simulink model "bus_roadtest_v3"  (R2018a)
settings: Solver=ode3  StartTime=0.0  StopTime=inf  FixedStep=0.01  RelTol=1e-3  EnableMultiTasking=on
PostLoadFcn:
  | , if any(exist('dsrtsu_mdlpostloadfcn', 'file') == [2, 3, 6]), try dsrtsu_mdlpostloadfcn('Execute', bdroot); catch fprintf('Error in PostLoadFcn (dsrtsu_mdlpostloadfcn) for model "%s":\n %s\n', bdroot, lasterr); end, end,
InitFcn:
  | bus_roadtest_v3_initial
values from neighbouring files (symbols this model uses):
  ay_max = 2    [Ini.m]
  delta_t = 0.01    [Ini.m]
  end_left_pass = 1    [Ini.m]
  end_right_pass = 0    [Ini.m]
  finish_node_id = length(Map_data(:,1))    [Ini.m]
  forward_length = 15    [Ini.m]
  gamma = sqrt(N_xaug+lambda)    [bus_roadtest_v3_initial.m]
  k_safe = 1    [Ini.m]
  nodes = nodes(1:index_node,:)    [Ini.m]
  rmin = 10    [Ini.m]
  segments = zeros(length(xy_ends_Pos(:,1)),3)    [Ini.m]
  start_node_id = 1    [Ini.m]
  Ts = 0.01    [bus_roadtest_v3_initial.m]
  Veh_CG = [0.5, 0.2]    [Ini.m]
  Veh_size = [1.99986,6.09558]    [Ini.m]
  vmax = 6    [Ini.m]
  weight = [weight_0,weight_0_cov,weight_i]    [bus_roadtest_v3_initial.m]
undefined symbols (not defined in the file or in its folder): Brake_table, DiscIntNeverNeededParam, Map_data, R, REF_GPS_RFS, Steer_gain_table, T
libraries: rtican x71, simulink x26, rti1401lib_adc_type4 x8, rti1401lib_dio_type4 x1
(part 18 of 18)

== matlab function bus_roadtest_v3/Target_planner/EndPointDecision1 ==
  data: x input; y input; End_x output; Path_x_0 input size=length(nodes(:,1)); Path_y_0 input size=length(nodes(:,1)); forward_length input; End_y output; path_length output
function [End_x,End_y,path_length] = EndPointDecision(x,y,Path_x_0,Path_y_0,forward_length)

% x = Vehicle_state(1,1); %vehicle global coordinate
% y = Vehicle_state(2,1);

Path_x = Path_x_0;
Path_y = Path_y_0;

%% Target plan
Path_RES_0 = zeros(20000,2);
Path_RES_0_1 = zeros(20000,2);
Res = 0.1;
count = 0;
count_1 = 0;
break_count = 0;
target_k = floor(forward_length/Res);

%找出切成10公分之投影點
Length_1 = ((Path_x(2)-Path_x(1))^2+(Path_y(2)-Path_y(1))^2)^0.5;
ang_1 = atan2(Path_y(2)-Path_y(1),Path_x(2)-Path_x(1));
if Length_1 > Res
    for j = 1:round(Length_1/Res)
        Path_RES_0_1(j,1) = Path_x(1) + (j-1)*Res*cos(ang_1);
        Path_RES_0_1(j,2) = Path_y(1) + (j-1)*Res*sin(ang_1);
        count_1 = j;
    end
else
    Path_RES_0_1(1,1) = Path_x(1);
    Path_RES_0_1(1,2) = Path_y(1);
    count_1 = 1;
end
Path_RES_1 = Path_RES_0_1((1:count_1),:);
ob_distance = (x-Path_RES_1(:,1)).^2 + (y - Path_RES_1(:,2)).^2;
[none,v_i] = min(ob_distance);
x_ob = Path_RES_1(v_i,1);
y_ob = Path_RES_1(v_i,2);
o_i = count_1-v_i;

if numel(Path_x(:,1))-2 >=1
    for i = 1:numel(Path_x(:,1))-2
        k = i+1;
        if break_count == 0
            Length = ((Path_x(k+1)-Path_x(k))^2+(Path_y(k+1)-Path_y(k))^2)^0.5;
            ang = atan2(Path_y(k+1)-Path_y(k),Path_x(k+1)-Path_x(k));
            if Length >= Res
                index_j = round(Length/Res);
                for j = 1:index_j
                    Path_RES_0(j+count,1) = Path_x(k) + (j-1)*Res*cos(ang);
                    Path_RES_0(j+count,2) = Path_y(k) + (j-1)*Res*sin(ang);
                end
                count = count + index_j;
%                 clear index_j;
            else
                Path_RES_0(1+count,1) = Path_x(k);
                Path_RES_0(1+count,2) = Path_y(k);
                count = count + 1;
            end
            if count > target_k - o_i
                break_count = 1;
            end
            target_forward_i = k;
        end
    end
else
    Path_RES_0 = [];
    count = 0;
end

temp = target_k+v_i;
if isempty(Path_RES_0) == 1
    if temp <= length(Path_RES_1(:,1))
        Path_RES = Path_RES_1(v_i:temp,:);
        End_x = Path_RES(target_k,1);% global
        End_y = Path_RES(target_k,2);
        case_1 = 1;
        path_length = target_k*0.1;
    else
        Path_RES = Path_RES_1(v_i:end,:);
        End_x = Path_RES(end,1);% global
        End_y = Path_RES(end,2);
        case_1 = 2;
        path_length = length(Path_RES)*0.1;
    end
else
    Path_RES = [Path_RES_1(v_i:end,:);Path_RES_0((1:count),:)];
    if target_k-o_i <= count
        End_x = Path_RES(target_k,1);% global
        End_y = Path_RES(target_k,2);
        case_1 = 3;
        path_length = target_k*0.1;
    else
        End_x = Path_RES(count+o_i,1);% global
        End_y = Path_RES(count+o_i,2);
        case_1 = 4;
        path_length = (count+o_i)*0.1;
    end
end

== matlab function bus_roadtest_v3/Target_planner/Final_Static_Path ==
  data: Map_data input; Static_Path_x output size=length(nodes(:,1)); Static_Path_y output size=length(nodes(:,1)); Static_Path_0 output size=size(Map_data); onoff input; dist_new input; dist_out output; path_new input size=length(nodes(:,1)); nodes input; dist_in input; path_out output size=length(nodes(:,1))
function [Static_Path_x,Static_Path_y,Static_Path_0,dist_out,path_out] = fcn(Map_data,onoff,dist_new,path_new,nodes,dist_in)

persistent path_out1
if isempty(path_out1)
    if onoff > 0
        path_out1 = path_new;
    else
        path_out1 = [0;0];
    end
end

if onoff > 0
    path_out1 = path_new;
end
path_out = path_out1;

if onoff > 0
    dist_out = dist_new;
else
    dist_out = dist_in;
end

Static_Path = zeros(length(path_out),3);
for i = 1 : length(path_out)
    Static_Path(i,:) = nodes(path_out(i),:);
end
Static_Path_x = Static_Path(:,2);
Static_Path_y = Static_Path(:,3);

xy_ends_static = [Static_Path(1:end-1,2) Static_Path(1:end-1,3) Static_Path(2:end,2) Static_Path(2:end,3)];
Static_segid_index = zeros(length(xy_ends_static(:,1)),1);
for i = 1 : length(xy_ends_static(:,1))
    Static_segid_index(i) = find((Map_data(:,2) == xy_ends_static(i,1))&(Map_data(:,3) == xy_ends_static(i,2))&(Map_data(:,4) == xy_ends_static(i,3))&(Map_data(:,5) == xy_ends_static(i,4)));
end
Static_Path_0 = zeros(length(xy_ends_static(:,1)),length(Map_data(1,:)));
for j = 1 : length(xy_ends_static(:,1))
    Static_Path_0(j,:) = Map_data(Static_segid_index(j),:);
end

Static_Path_0 = Map_data;

== matlab function bus_roadtest_v3/Target_planner/Forward_Length_Decision ==
  data: Car_velocity input; Forward_length_final output; LAS0 input; LAT input; Forward_length input; op_dist input; seg_LaneWidth input; forwardendheading0 input; Rotz input; avoidancemode input; Intrusion_range input; Path_flag input; diffheading1 output; forward_check_i input; forward_check_o output
function [Forward_length_final,diffheading1,forward_check_o] = fcn(Car_velocity,LAS0,LAT,Forward_length,op_dist,seg_LaneWidth,forwardendheading0,Rotz,avoidancemode,Intrusion_range,Path_flag,forward_check_i)

diffheading = abs(forwardendheading0 - Rotz);
if diffheading > 180
    diffheading1 = abs(diffheading - 360);
else
    diffheading1 = diffheading;
end

if forward_check_i == 1
    if diffheading1 > 10 || op_dist > seg_LaneWidth/4
        Switch = 1;
    else
        Switch = 0;
    end
else
    if avoidancemode == 1
        Switch = 0;
    else
        if diffheading1 > 45 % || op_dist > seg_LaneWidth/2
            Switch = 1;
        else
            Switch = 0;
        end
    end
end

% if Switch == 1
%     Forward_length_final = Car_velocity*LAT + LAS0;
%     forward_check_o = 1;
% else
%     Forward_length_final = Forward_length;
%     forward_check_o = 0;
% end

% Path_flag_current = Path_flag;
% if Path_flag_last - Path_flag_current == -1
%     range = Intrusion_range + 0.5;
% else
%     range = range_last;
% end

if Switch == 1
    Forward_length_final = Car_velocity*LAT + LAS0;
    forward_check_o = 1;
else
    if Path_flag == 0
%         Forward_length_final = Forward_length;
        Forward_length_final = Car_velocity*LAT + LAS0;
    else
%         Forward_length_final = Forward_length;
        Forward_length_final = Intrusion_range;
    end
    forward_check_o = 0;
end

== matlab function bus_roadtest_v3/Target_planner/Forward_Seg ==
  data: Static_Path_0 input size=size(Map_data); Forward_Static_Path_x output size=length(nodes(:,1)); Vehicle_state input; SEG_ID_NEAR_TRUE input; Car_Velocity input; forward_length input; Forward_Static_Path_y output size=length(nodes(:,1)); Forward_Static_Path_id output size=length(nodes(:,1)); start_ind_out output; seg_id output size=size(Map_data(:,1)); end_seg_id output; case_0 output; end_ind output
function [Forward_Static_Path_x,Forward_Static_Path_y,Forward_Static_Path_id,start_ind_out,seg_id,end_seg_id,case_0,end_ind]= FowardSeg(Static_Path_0,Vehicle_state,SEG_ID_NEAR_TRUE,Car_Velocity,forward_length)

Static_Path = Static_Path_0;

x = Vehicle_state(1,1); %vehicle global coordinate
y = Vehicle_state(2,1);

xy_ends_POS = Static_Path(:,2:5);
seg_id = Static_Path(:,1);
seg_length = Static_Path(:,9);

if xy_ends_POS(1,1) == xy_ends_POS(end,3) && xy_ends_POS(1,2) == xy_ends_POS(end,4)
    Static_PathCycle = 1;
else
    Static_PathCycle = 0;
end

[~,start_ind] = max(seg_id(:) == SEG_ID_NEAR_TRUE);
% start_ind = find(seg_id(:) == SEG_ID_NEAR_TRUE);
start_ind_out = start_ind(1);
% 加入從長度判定要幾個seg 預計至少20m
total_length = ((x-xy_ends_POS(start_ind(1),3))^2+(y-xy_ends_POS(start_ind(1),4))^2)^0.5;
end_ind_0 = start_ind(1);
case_0 = 0;
end_ind = 0;
for i = 1 : length(seg_length)
    if total_length > forward_length
        end_ind = end_ind_0;
        break;
    end
    if (start_ind(1)+i) <= length(seg_length)
        total_length = total_length + seg_length(start_ind(1)+i);
        end_ind_0 = start_ind(1)+i;
        case_0 = 1;
    else
        if Static_PathCycle == 1
            total_length = total_length + seg_length(start_ind(1)+i-length(seg_length));
            end_ind_0 = start_ind(1)+i - length(seg_length);
            case_0 = 2;
        else
            total_length = total_length;
            end_ind = end_ind_0;
            case_0 = 3;
            break;
        end
    end
end

Forward_Static_Path_id_0 = zeros(length(seg_id),1);
if isempty(start_ind) == 1
    start_ind(1) = 1;
    end_ind = length(seg_id(:));
    Static_Path_ends_POS = xy_ends_POS(start_ind(1):end_ind(1),:);
    Forward_Static_Path_id_0(:) = seg_id(:);
    Forward_Static_Path_length = length(seg_id(:));
else
    if case_0 == 1 || case_0 == 0
        Static_Path_ends_POS = xy_ends_POS(start_ind(1):end_ind(1),:);
        Forward_Static_Path_id_0(1:(end_ind(1)-start_ind(1)+1)) = seg_id(start_ind(1):end_ind(1));
        Forward_Static_Path_length = length(seg_id(start_ind(1):end_ind(1)));
    else
        if case_0 == 2
            Static_Path_ends_POS = [xy_ends_POS(start_ind(1):end,:);xy_ends_POS(1:end_ind(1),:)];
            Forward_Static_Path_id_0(1:(1+length(seg_id(:))-start_ind(1)+end_ind(1))) = [seg_id(start_ind(1):end);seg_id(1:end_ind(1))];
            Forward_Static_Path_length = length([seg_id(start_ind(1):end);seg_id(1:end_ind(1))]);
        else
            end_ind = length(seg_id(:));
            Static_Path_ends_POS = xy_ends_POS(start_ind(1):end_ind(1),:);
            Forward_Static_Path_id_0(1:end_ind(1)-start_ind(1)+1) = seg_id(start_ind(1):end_ind(1));
            Forward_Static_Path_length = length(seg_id(start_ind(1):end_ind(1)));
        end
    end
end

Forward_Static_Path_id = Forward_Static_Path_id_0(1:Forward_Static_Path_length);

Forward_Static_Path = zeros(length(Static_Path_ends_POS(:,1))+1,2);
Forward_Static_Path(1:length(Static_Path_ends_POS(:,1)),1:2) = Static_Path_ends_POS(:,1:2);
Forward_Static_Path(length(Static_Path_ends_POS(:,1))+1,1:2) = Static_Path_ends_POS(length(Static_Path_ends_POS(:,1)),3:4);

Forward_Static_Path_x = Forward_Static_Path(1:numel(Forward_Static_Path(:,1)),1);
Forward_Static_Path_y = Forward_Static_Path(1:numel(Forward_Static_Path(:,1)),2);

end_seg_id = Forward_Static_Path_id(end);

% Forward_Static_Path_id = seg_id(start_ind_out:end);
% Forward_Static_Path_x = [xy_ends_POS(start_ind_out:end,1);xy_ends_POS(end,3)];
% Forward_Static_Path_y = [xy_ends_POS(start_ind_out:end,2);xy_ends_POS(end,4)];

== matlab function bus_roadtest_v3/Target_planner/Forward_Seg1 ==
  data: Static_Path_0 input size=size(Map_data); Forward_Static_Path_x output size=length(nodes(:,1)); Vehicle_state input; SEG_ID_NEAR_TRUE input; Car_Velocity input; forward_length input; Forward_Static_Path_y output size=length(nodes(:,1)); Forward_Static_Path_id output size=length(nodes(:,1))
function [Forward_Static_Path_x,Forward_Static_Path_y,Forward_Static_Path_id]= FowardSeg(Static_Path_0,Vehicle_state,SEG_ID_NEAR_TRUE,Car_Velocity,forward_length)

Static_Path = Static_Path_0;

x = Vehicle_state(1,1); %vehicle global coordinate
y = Vehicle_state(2,1);

xy_ends_POS = Static_Path(:,2:5);
seg_id = Static_Path(:,1);
seg_length = Static_Path(:,9);

if xy_ends_POS(1,1) == xy_ends_POS(end,3) && xy_ends_POS(1,2) == xy_ends_POS(end,4)
    Static_PathCycle = 1;
else
    Static_PathCycle = 0;
end

[~,start_ind] = max(seg_id(:) == SEG_ID_NEAR_TRUE);
% start_ind = find(seg_id(:) == SEG_ID_NEAR_TRUE);
start_ind_out = start_ind(1);
% 加入從長度判定要幾個seg 預計至少20m
total_length = ((x-xy_ends_POS(start_ind(1),3))^2+(y-xy_ends_POS(start_ind(1),4))^2)^0.5;
end_ind_0 = start_ind(1);
case_0 = 0;
end_ind = 0;
for i = 1 : length(seg_length)
    if total_length > forward_length
        end_ind = end_ind_0;
        break;
    end
    if (start_ind(1)+i) <= length(seg_length)
        total_length = total_length + seg_length(start_ind(1)+i);
        end_ind_0 = start_ind(1)+i;
        case_0 = 1;
    else
        if Static_PathCycle == 1
            total_length = total_length + seg_length(start_ind(1)+i-length(seg_length));
            end_ind_0 = start_ind(1)+i - length(seg_length);
            case_0 = 2;
        else
            total_length = total_length;
            end_ind = end_ind_0;
            case_0 = 3;
            break;
        end
    end
end

Forward_Static_Path_id_0 = zeros(length(seg_id),1);
if isempty(start_ind) == 1
    start_ind(1) = 1;
    end_ind = length(seg_id(:));
    Static_Path_ends_POS = xy_ends_POS(start_ind(1):end_ind(1),:);
    Forward_Static_Path_id_0(:) = seg_id(:);
    Forward_Static_Path_length = length(seg_id(:));
else
    if case_0 == 1 || case_0 == 0
        Static_Path_ends_POS = xy_ends_POS(start_ind(1):end_ind(1),:);
        Forward_Static_Path_id_0(1:(end_ind(1)-start_ind(1)+1)) = seg_id(start_ind(1):end_ind(1));
        Forward_Static_Path_length = length(seg_id(start_ind(1):end_ind(1)));
    else
        if case_0 == 2
            Static_Path_ends_POS = [xy_ends_POS(start_ind(1):end,:);xy_ends_POS(1:end_ind(1),:)];
            Forward_Static_Path_id_0(1:(1+length(seg_id(:))-start_ind(1)+end_ind(1))) = [seg_id(start_ind(1):end);seg_id(1:end_ind(1))];
            Forward_Static_Path_length = length([seg_id(start_ind(1):end);seg_id(1:end_ind(1))]);
        else
            end_ind = length(seg_id(:));
            Static_Path_ends_POS = xy_ends_POS(start_ind(1):end_ind(1),:);
            Forward_Static_Path_id_0(1:end_ind(1)-start_ind(1)+1) = seg_id(start_ind(1):end_ind(1));
            Forward_Static_Path_length = length(seg_id(start_ind(1):end_ind(1)));
        end
    end
end

Forward_Static_Path_id = Forward_Static_Path_id_0(1:Forward_Static_Path_length);

Forward_Static_Path = zeros(length(Static_Path_ends_POS(:,1))+1,2);
Forward_Static_Path(1:length(Static_Path_ends_POS(:,1)),1:2) = Static_Path_ends_POS(:,1:2);
Forward_Static_Path(length(Static_Path_ends_POS(:,1))+1,1:2) = Static_Path_ends_POS(length(Static_Path_ends_POS(:,1)),3:4);

Forward_Static_Path_x = Forward_Static_Path(1:numel(Forward_Static_Path(:,1)),1);
Forward_Static_Path_y = Forward_Static_Path(1:numel(Forward_Static_Path(:,1)),2);

end_seg_id = Forward_Static_Path_id(end);

== matlab function bus_roadtest_v3/Target_planner/Forward_Seg_0 ==
  data: Static_Path_0 input size=size(Map_data); Forward_Static_Path_heading output; Vehicle_state input; SEG_ID_NEAR_TRUE input; forward_length input
function Forward_Static_Path_heading = FowardSeg(Static_Path_0,Vehicle_state,SEG_ID_NEAR_TRUE,forward_length)

Static_Path = Static_Path_0;

x = Vehicle_state(1,1); %vehicle global coordinate
y = Vehicle_state(2,1);

xy_ends_POS = Static_Path(:,2:5);
seg_id = Static_Path(:,1);
seg_length = Static_Path(:,9);

if xy_ends_POS(1,1) == xy_ends_POS(end,3) && xy_ends_POS(1,2) == xy_ends_POS(end,4)
    Static_PathCycle = 1;
else
    Static_PathCycle = 0;
end

[~,start_ind] = max(seg_id(:) == SEG_ID_NEAR_TRUE);
% start_ind = find(seg_id(:) == SEG_ID_NEAR_TRUE);
start_ind_out = start_ind(1);
% 加入從長度判定要幾個seg 預計至少20m
total_length = ((x-xy_ends_POS(start_ind(1),3))^2+(y-xy_ends_POS(start_ind(1),4))^2)^0.5;
end_ind_0 = start_ind(1);
case_0 = 0;
end_ind = 0;
for i = 1 : length(seg_length)
    if total_length > forward_length
        end_ind = end_ind_0;
        break;
    end
    if (start_ind(1)+i) <= length(seg_length)
        total_length = total_length + seg_length(start_ind(1)+i);
        end_ind_0 = start_ind(1)+i;
        case_0 = 1;
    else
        if Static_PathCycle == 1
            total_length = total_length + seg_length(start_ind(1)+i - length(seg_length));
            end_ind_0 = start_ind(1)+i - length(seg_length);
            case_0 = 2;
        else
            total_length = total_length;
            end_ind = end_ind_0;
            case_0 = 3;
            break;
        end
    end
end

Forward_Static_Path_id_0 = zeros(length(seg_id),1);
if isempty(start_ind) == 1
    start_ind(1) = 1;
    end_ind = length(seg_id(:));
    Forward_Static_Path_id_0(:) = seg_id(:);
    Forward_Static_Path_length = length(seg_id(:));
else
    if case_0 == 1 || case_0 == 0
        Forward_Static_Path_id_0(1:(end_ind(1)-start_ind(1)+1)) = seg_id(start_ind(1):end_ind(1));
        Forward_Static_Path_length = length(seg_id(start_ind(1):end_ind(1)));
    else
        if case_0 == 2
            Forward_Static_Path_id_0(1:(1+length(seg_id(:))-start_ind(1)+end_ind(1))) = [seg_id(start_ind(1):end);seg_id(1:end_ind(1))];
            Forward_Static_Path_length = length([seg_id(start_ind(1):end);seg_id(2:end_ind(1))]);
        else
            end_ind = length(seg_id(:));
            Forward_Static_Path_id_0(1:end_ind(1)-start_ind(1)+1) = seg_id(start_ind(1):end_ind(1));
            Forward_Static_Path_length = length(seg_id(start_ind(1):end_ind(1)));
        end
    end
end

Forward_Static_Path_id = Forward_Static_Path_id_0(1:Forward_Static_Path_length);

[~,ind] = max(Static_Path(:,1) == Forward_Static_Path_id(end));
Forward_Static_Path_heading = Static_Path(ind,8);

== matlab function bus_roadtest_v3/Target_planner/MATLAB Function ==
  data: Vehicle_state input; Vehicle_nextstep output; Veh_Velocity input; LAS0 input; LAT input; XP_final input; YP_final input; L_path_fianl input; Vehicle_Target_x output size=1; Vehicle_Target_y output size=1; TargetXY output size=[2 1]; Detour_flag input
function [Vehicle_nextstep,Vehicle_Target_x,Vehicle_Target_y,TargetXY]  = fcn(Vehicle_state,Veh_Velocity,LAS0,LAT,XP_final,YP_final,L_path_fianl,Detour_flag)
%% Next Step Position
% u_final = Veh_Velocity*delta_t/L_path(Jminind);
% u_final_1 = u_final-0.001;
% if Detour_flag == 1%% && Veh_Velocity < 1.5
%     u_final_Target = 1;
% else
    u_final_Target = (Veh_Velocity*LAT+LAS0)/L_path_fianl;
% end
% x_nextstep = XP_final(1) + XP_final(2)*u_final + XP_final(3)*u_final^2 + XP_final(4)*u_final^3 + XP_final(5)*u_final^4 + XP_final(6)*u_final^5;
% y_nextstep = YP_final(1) + YP_final(2)*u_final + YP_final(3)*u_final^2 + YP_final(4)*u_final^3 + YP_final(5)*u_final^4 + YP_final(6)*u_final^5;
% x_nextstep_1 = XP_final(1) + XP_final(2)*u_final_1 + XP_final(3)*u_final_1^2 + XP_final(4)*u_final_1^3 + XP_final(5)*u_final_1^4 + XP_final(6)*u_final_1^5;
% y_nextstep_1 = YP_final(1) + YP_final(2)*u_final_1 + YP_final(3)*u_final_1^2 + YP_final(4)*u_final_1^3 + YP_final(5)*u_final_1^4 + YP_final(6)*u_final_1^5;
x_target = XP_final(1) + XP_final(2)*u_final_Target + XP_final(3)*u_final_Target^2 + XP_final(4)*u_final_Target^3 + XP_final(5)*u_final_Target^4 + XP_final(6)*u_final_Target^5;
y_target = YP_final(1) + YP_final(2)*u_final_Target + YP_final(3)*u_final_Target^2 + YP_final(4)*u_final_Target^3 + YP_final(5)*u_final_Target^4 + YP_final(6)*u_final_Target^5;
n = 0.02;
% heading
% if x_nextstep == x_nextstep_1
%    SLOPE_tonext = inf; % s_i is a vertical line
% else
%    SLOPE_tonext = (y_nextstep-y_nextstep_1)/(x_nextstep-x_nextstep_1);
% end
% if SLOPE_tonext == inf
%     if y_nextstep-y_nextstep_1 > 0
%         heading_nextstep_0 = pi/2;
%     else
%         heading_nextstep_0 = -pi/2;
%     end
% else
%     heading_nextstep_0 = atan(SLOPE_tonext);
% end
% if x_nextstep-x_nextstep_1 >= 0
%     heading_nextstep_1 = heading_nextstep_0 - pi/2; %along
% else
%     heading_nextstep_1 = heading_nextstep_0 + pi/2; %along 
% end
% heading_nextstep = (heading_nextstep_1-3*pi/2)*180/pi;
% while heading_nextstep < 0
%     heading_nextstep = heading_nextstep + 360;
% end
% if x_target == x_nextstep
%    SLOPE_targettonext = inf; % s_i is a vertical line
% else
%    SLOPE_targettonext = (y_target-y_nextstep)/(x_target-x_nextstep);
% end
% if SLOPE_targettonext == inf
%     if y_target-y_nextstep > 0
%         heading_target_0 = pi/2;
%     else
%         heading_target_0 = -pi/2;
%     end
% else
%     heading_target_0 = atan(SLOPE_targettonext);
% end
% if x_target-x_nextstep >= 0
%     heading_target_1 = heading_target_0 - pi/2; %along
% else
%     heading_target_1 = heading_target_0 + pi/2; %along 
% end
% heading_target = (heading_target_1-3*pi/2)*180/pi;
% while heading_target < 0
%     heading_target = heading_target + 360;
% end
% if heading_target-heading_nextstep > 180
%     heading_target = heading_target - 360;
%     final_heading = heading_target*n + heading_nextstep*(1-n);
% elseif heading_target-heading_nextstep < -180
%     heading_target = heading_target + 360;
%     final_heading = heading_target*n + heading_nextstep*(1-n);
% else
%     final_heading = heading_target*n + heading_nextstep*(1-n);
% end
Vehicle_nextstep = Vehicle_state;
TargetXY = [x_target;y_target];

%% vehicle target x y
heading = Vehicle_state(3,1);
rotate_ang = -heading;
Vehicle_Target = [cos(rotate_ang),-sin(rotate_ang);sin(rotate_ang),cos(rotate_ang)]*[x_target-Vehicle_state(1,1);y_target-Vehicle_state(2,1)];
Vehicle_Target_x = Vehicle_Target(1);
Vehicle_Target_y = Vehicle_Target(2);

== matlab function bus_roadtest_v3/Target_planner/MM ==
  data: seg_id_near output; Map_data input size=size(Map_data); Position_X input; op_distance output; Oi_near output; num_lane_direction output; seg_heading output; seg_LaneWidth output; Postion_Y input; Position_H input; seg_Curvature output; note output
function [seg_id_near,op_distance,Oi_near,num_lane_direction,seg_heading,seg_LaneWidth,seg_Curvature,note]= fcn(Map_data,Position_X,Postion_Y,Position_H)

%%% Map_data=[Seg_XY SLOPE_SEG SHIFT_SEG Heading_X LENGTH_SEG]; nx8
XY_ID=Map_data(:,1);
XY_INI=Map_data(:,2:3);
XY_END=Map_data(:,4:5);
SLOPE_SEG=Map_data(:,6);
SHIFT_SEG=Map_data(:,7);
HEADING_DIFFERENCE_VEH_ROAD = 45*pi/180;
DIST_THREAD_5 = 4;

m=length(XY_ID);
oi_xy=zeros(m,2);
dist_op=zeros(m,1);
for i =1:m
    if SLOPE_SEG(i) == inf
        oi_xy(i,1) = XY_INI(i,1); % x position of the projection point on this segment
        oi_xy(i,2) = Postion_Y;
    elseif SLOPE_SEG(i)==0
        oi_xy(i,1) = Position_X;
        oi_xy(i,2) = XY_INI(i,2);
    else
        a_j = -1/SLOPE_SEG(i);
        b_j = Postion_Y - a_j*Position_X;
        oi_xy(i,1) = (b_j-SHIFT_SEG(i))/(SLOPE_SEG(i)-a_j); % x position of the i-th projection point
        oi_xy(i,2) = (SLOPE_SEG(i)*b_j - a_j*SHIFT_SEG(i))/(SLOPE_SEG(i)-a_j); % y position of the i-th projection point 
    end          
end

for i = 1:length(oi_xy(:,1))
    dist_op(i,1)=sqrt((oi_xy(i,1)-Position_X)^2+(oi_xy(i,2)-Postion_Y)^2);     
end

[seg_id_near,op_distance,oi_near,note,seg_direction,head_err,num_lane_direction,seg_heading] = MM(Position_H*180/pi,[Position_X;Postion_Y],oi_xy,dist_op,Map_data,HEADING_DIFFERENCE_VEH_ROAD,DIST_THREAD_5);
Oi_near=oi_near';
[~,seg_id_ind] = max(XY_ID == seg_id_near);
seg_LaneWidth = Map_data(seg_id_ind,11);
seg_Curvature = Map_data(seg_id_ind,14);

%% MM function
function [seg_id_near,op_distance,oi_near,note,seg_direction,head_err,num_lane_direction,seg_heading] = MM(heading,X_pos,oi_xy,dist_op,Map_data,HEADING_DIFFERENCE_VEH_ROAD,DIST_THREAD_5)
note=0;
seg_id_near=double(0);
op_distance=0;
oi_near=zeros(1,2);
end_pt=zeros(1,2);
seg_direction=0;
[dist_sort,index] = sort(dist_op);
index=[index,zeros(length(index),1)];

xy_ini = Map_data(:,2:3);
xy_end = Map_data(:,4:5);
SLOPE_SEG = Map_data(:,6);
seg_id = Map_data(:,1);
LENGTH_SEG = Map_data(:,9);
SEG_GPS_HEAD = Map_data(:,8);
SEG_GPS_HEAD=[seg_id SEG_GPS_HEAD];

%%    Map Matching

for j = 1:length(xy_ini(:,1));
    i = index(j,1);
    dis_temp1 = sqrt((xy_ini(i,1)-oi_xy(i,1))^2+(xy_ini(i,2)-oi_xy(i,2))^2);
    dis_temp2 = sqrt((xy_end(i,1)-oi_xy(i,1))^2+(xy_end(i,2)-oi_xy(i,2))^2);
 
    if (dis_temp1 <= LENGTH_SEG(i)&& dis_temp2 <= LENGTH_SEG(i));
        index(j,2) = 1; %oi_xy lies in between xy_ini and xy_end
    else index(j,2) = 0;
    end
end

%"possible_seg" contains the sequence of possible segment index
ind_temp = find(index(1:end,2)==1);
% ind_temp=ind_temp(1);
if isempty(ind_temp);
   note = 1;  % 1: the projection point is not between two segment ends for any road segment;
              % search nearest segment by finding the nearest segment end!             
   %compare distances between ends and X_pos!     
    dist_ini = rel_dist_xy(X_pos,xy_ini);
    dist_end = rel_dist_xy(X_pos,xy_end);
  
    [min_dis_ini,junk1] = min(dist_ini);   %-------------------------------------------------哪來的junk 1 &2 ?
    [min_dis_end,junk2] = min(dist_end);
    if min_dis_ini<= min_dis_end; %X_pos is closer to the end
       possible_seg = junk1; %index
       end_pt = xy_ini(junk1,1:end);
    else 
       possible_seg = junk2; %index
       end_pt = xy_end(junk2,1:end);
    end

    seg_id_near = seg_id(possible_seg);
    
    op_distance = dist_op(possible_seg);
    oi_near = oi_xy(possible_seg,1:2);
    if possible_seg>1 && possible_seg<length(seg_id)
    op_distance_n=rel_dist_xy(X_pos,oi_near);
    min_ini_pos=rel_dist_xy(X_pos,xy_ini(possible_seg,:));
    min_end_pos=rel_dist_xy(X_pos,xy_end(possible_seg,:));
    if op_distance_n<min_ini_pos && op_distance_n<min_end_pos
        note = 0;
    else
        note = 1;
    end
    else
        op_distance_n=rel_dist_xy(X_pos,oi_near);
        min_ini_pos=rel_dist_xy(X_pos,xy_ini(possible_seg,:));
        min_end_pos=rel_dist_xy(X_pos,xy_end(possible_seg,:));
    end
    
%    seg_direction = Get_Seg_Heading(seg_id_near,heading);
%    %%%不用老師程式--
    temp_ind = find(SEG_GPS_HEAD(:,1) == seg_id_near);
    head_err = abs(heading-SEG_GPS_HEAD(temp_ind(1),2)); 
    if head_err <= HEADING_DIFFERENCE_VEH_ROAD
    seg_direction = 1; %1= along slope, 2:adverse
    elseif head_err>=HEADING_DIFFERENCE_VEH_ROAD && head_err<=90
    seg_direction = 0; %unknown
    else
    seg_direction = 2;
    end
%     %%%不用老師程式--
 elseif length(ind_temp(1)) ==1; %only 
%      find one segment candidate
       note = 0; % 0: the projection point lies between two ends of each segment    
       possible_seg = index(ind_temp(1),1);
       seg_id_near = seg_id(possible_seg);
       op_distance = dist_op(possible_seg);
       oi_near = oi_xy(possible_seg,1:2);
       end_pt = [0,0]; % temp./unused nominal values
%      seg_direction = Get_Seg_Heading(seg_id_near,heading); %get road segment heading direction

        temp_ind = find(SEG_GPS_HEAD(:,1) == seg_id_near);
        head_err = abs(heading-SEG_GPS_HEAD(temp_ind(1),2)); 
       if head_err <= HEADING_DIFFERENCE_VEH_ROAD;
            seg_direction = 1; %1= along slope, 2:adverse
       elseif head_err>=HEADING_DIFFERENCE_VEH_ROAD && head_err<=90
            seg_direction = 0; %unknown
       else
            seg_direction = 2;
       end
       %Now compare the distances between X_pos and all segment ends with
       %op_distance. If find closer node, may discard previous found segment.
       
       dist_ini = rel_dist_xy(X_pos,xy_ini);
       dist_end = rel_dist_xy(X_pos,xy_end);
           %dis_min = min(dist_ini,dist_end);
           %dis_min_val = min(dis_min);
           %temp_a = find(dis_min == dis_min_val); % diff, segments may have the same node!
       [min_dis_ini,junk1] = min(dist_ini);
       [min_dis_end,junk2] = min(dist_end);
       dis_min_val = min(min_dis_ini,min_dis_end);
       
    if dis_min_val < op_distance;%min(op_distance); %X_pos is closer to one of the segment ends than its project point         
       note = 2; %Change the "note" value! 
                 %special case: the found projection pt. (oi_near) lie(s) between two ends 
                 %of one segment, but the associated segments may not
                 %the nearest road segments.          
       %search the nearest node of road segments. 
        if min_dis_ini<= min_dis_end;
           temp_a = junk1;
           end_pt = xy_ini(junk1,1:end);
        else 
           temp_a = junk2;
           end_pt = xy_end(junk2,1:end);
        end
       
        
        if length(temp_a)>1; %multiple segment case
            
           seg_head_pos = SEG_GPS_HEAD(temp_a,2); %road segment heading in the positive slope direction
%            seg_head_neg = SEG_GPS_HEAD(temp_a,3);
           
           %find smallest heading discrepancy in positive slope direction
           [junk1,ind_pos] = min(abs(heading - seg_head_pos(1:end)));
               
           %find smallest heading discrepancy in negative/adverse slope direction
%            [junk2,ind_neg] = min(abs(angle_convert(heading - seg_head_neg(1:end))));
           
           %compare two smallest heading erros of two adverse directions
 
              ind = temp_a(ind_pos);
              seg_id_near = seg_id(ind);
              op_distance = dist_op(ind);
              oi_near = oi_xy(ind,1:2);
              temp_ind = find(SEG_GPS_HEAD(:,1) == seg_id_near);
              head_err = abs(heading-SEG_GPS_HEAD(temp_ind(1),2)); 

              if head_err <= HEADING_DIFFERENCE_VEH_ROAD;
                    seg_direction = 1; %1= along slope, 2:adverse
              elseif head_err>=HEADING_DIFFERENCE_VEH_ROAD && head_err<=90
                    seg_direction = 0; %unknown
              else
                    seg_direction = 2;
              end
       
        else %single segment case
              temp_ind = find(SEG_GPS_HEAD(:,1) == seg_id_near);
              head_err = abs(heading-SEG_GPS_HEAD(temp_ind(1),2)); 

              if head_err <= HEADING_DIFFERENCE_VEH_ROAD;
                    seg_direction = 1; %1= along slope, 2:adverse
              elseif head_err>=HEADING_DIFFERENCE_VEH_ROAD && head_err<=90
                    seg_direction = 0; %unknown
              else
                    seg_direction = 2;
              end
                 seg_id_near = seg_id(temp_a);
                 op_distance = dist_op(temp_a);
                 oi_near = oi_xy(temp_a,1:2);
        end
    end
 else %multiple segment candidates
       note = 0; % 0: the projection point lies between two ends of each segment          
       cand_seg = index(ind_temp,1);
       %cand_id = seg_id(cand_seg(1:2)); % only check the first two colsest segment candidate
       cand_op_dist = dist_op(cand_seg(1:2));
       
       %find road heading for the first two candidates
        head_pos = SEG_GPS_HEAD(cand_seg(1:2),2);

       %first candidate
        err_1 =  abs(heading - head_pos(1));
        %temp = [head_pos(1),head_neg(1)];
        %cand_head(1) = temp(ii);
        %clear ii;
       %second candidate
        err_2 = abs(heading - head_pos(2));
        %temp = [head_pos(2),head_neg(2)];
        %cand_head(2) = temp(ii);
        %clear ii;
        
       %compare two heading errors
        if err_1<= err_2 && err_1< HEADING_DIFFERENCE_VEH_ROAD; % HEADING_DIFFERENCE_VEH_ROAD = 45/180*pi
           possible_seg =  cand_seg(1);
           seg_direction = 1;
        elseif err_2< err_1 && ((cand_op_dist(2)-cand_op_dist(1))< DIST_THREAD_5); %DIST_THREAD_5 = 9 m
           possible_seg = cand_seg(2); 
           seg_direction = 2;
        else
           possible_seg = cand_seg(1);
           seg_direction = 1;
        end
        
       clear err_1 err_2 cand_op_dist cand_seg head_pos head_neg direction_1 direction_2;
       %possible_seg = index(ind_temp,1);       
       seg_id_near = seg_id(possible_seg);
       op_distance = dist_op(possible_seg);
       oi_near = oi_xy(possible_seg,1:2);
       end_pt = [0,0]; % temp./unused nominal values
        
       %Now compare the distances between X_pos and all segment ends with
       %above op_distance.
       %compute distances between X_pos and all segment ends
       dist_ini = rel_dist_xy(X_pos,xy_ini);
       dist_end = rel_dist_xy(X_pos,xy_end);
           %dis_min = min(dist_ini,dist_end);
           %dis_min_val = min(dis_min);
           %temp_a = find(dis_min == dis_min_val); % diff, segments may have the same node!
       [min_dis_ini,junk1] = min(dist_ini);
       [min_dis_end,junk2] = min(dist_end);
       dis_min_val = min(min_dis_ini,min_dis_end); 
       
    if dis_min_val < op_distance; %min(op_distance); %X_pos is closer to one of the segment ends than its project point         
       note = 2; %Change the note value! 
                 %special case: the found projection pt. (oi_near) lie(s) between two ends 
                 %of one segment, but the associated segments may not be
                 %the nearest road segments.          
       %search the nearest node of road segments. 
        if min_dis_ini<= min_dis_end;
           temp_a = junk1;
           end_pt = xy_ini(junk1,1:2);
        else 
           temp_a = junk2;
           end_pt = xy_end(junk2,1:2);
        end
        clear junk1 junk2;
        
        if length(temp_a)>1; %multiple segment case, then compare heading with road segment heading
          
           seg_head_pos = SEG_GPS_HEAD(temp_a,2);
           [junk1,ind_pos] = min(abs(heading - seg_head_pos(1:end)));


              ind = temp_a(ind_pos);
              seg_id_near = seg_id(ind);
              op_distance = dist_op(ind);
              oi_near = oi_xy(ind,1:2);

              temp_ind = find(SEG_GPS_HEAD(:,1) == seg_id_near);
              head_err = abs(heading-SEG_GPS_HEAD(temp_ind(1),2)); 

              if head_err <= HEADING_DIFFERENCE_VEH_ROAD;
                    seg_direction = 1; %1= along slope, 2:adverse
              elseif head_err>=HEADING_DIFFERENCE_VEH_ROAD && head_err<=90
                    seg_direction = 0; %unknown
              else
                    seg_direction = 2;
              end

       
        else %determine road direction is positive or negative slope direction

             seg_id_near = seg_id(temp_a);
             op_distance = dist_op(temp_a);
             oi_near = oi_xy(temp_a,1:2);
             temp_ind = find(SEG_GPS_HEAD(:,1) == seg_id_near);
              head_err = abs(heading-SEG_GPS_HEAD(temp_ind(1),2)); 

              if head_err <= HEADING_DIFFERENCE_VEH_ROAD;
                    seg_direction = 1; %1= along slope, 2:adverse
              elseif head_err>=HEADING_DIFFERENCE_VEH_ROAD && head_err<=90
                    seg_direction = 0; %unknown
              else
                    seg_direction = 2;
              end

        end
    end
           
end
%% check projection distance positive or negative Y=AX+B ;AX+B-Y>0 or AX+B-Y<0
Heading_X_rad = Map_data(:,8).*pi./180;
[~,temp_ind] = max(seg_id(:,1) == seg_id_near);
A=SLOPE_SEG(temp_ind);
B=oi_near(2)-A*oi_near(1);
if A < 0
    C=-A*X_pos(1)-B+X_pos(2);
    if Heading_X_rad(temp_ind) > 3*pi/2 && Heading_X_rad(temp_ind) < 2*pi
        C = C;
    else
        C = -C;
    end
elseif A == 0
    if oi_near(2)<X_pos(2)
        C=-1;
    else
        C=1;
    end
else
    C=A*X_pos(1)+B-X_pos(2);
    if Heading_X_rad(temp_ind) > pi && Heading_X_rad(temp_ind) < 3*pi/2
        C = C;
    else
        C = -C;
    end
end
if C<0 
    d=1;
elseif C==0
    d=1;
else
    d=-1;
end
num_lane_direction=[A;B;C;d];
seg_heading = Heading_X_rad(temp_ind);
%% rel_dist
function dist = rel_dist_xy(ref_xy,pt_xy)
% This function computes relative distances between given reference point, ref_xy, and positions, p_xy. 
% ref_xy = [x0,y0];
% pt_xy = [x,y];

temp = (pt_xy(:,1)-ref_xy(1)).^2 + (pt_xy(:,2)-ref_xy(2)).^2;
dist = temp.^0.5;

== matlab function bus_roadtest_v3/Target_planner/Target_Point_seg_info1 ==
  data: Map_data input; Target_seg_heading output; Target_seg_id input
function Target_seg_heading = fcn(Map_data,Target_seg_id)

if Target_seg_id > Map_data(:,1)
    Target_seg_id = length(Map_data(:,1));
end

Target_seg_heading = Map_data(Target_seg_id,8).*pi./180;

== matlab function bus_roadtest_v3/Target_planner/trajectory merge ==
  data: XP_final input; XP_final_2 output; YP_final input; XP_final_1 input; YP_final_1 input; Path_final input; Path_final_1 input; YP_final_2 output; Path_final_2 output
function [XP_final_2,YP_final_2,Path_final_2] = fcn(XP_final,YP_final,XP_final_1,YP_final_1,Path_final,Path_final_1)

XP_final_2 = [XP_final;XP_final_1];
YP_final_2 = [YP_final;YP_final_1];
Path_final_2 = [Path_final;Path_final_1(2:end,:)];

== matlab function bus_roadtest_v3/Speed_profile/High level controller/ACC/MATLAB Function ==
  data: Relative_distance input; cmd output; Reference_m input; Front_speed input; Speed_set input; AEB_range input; close_flag output
function [cmd , close_flag] = fcn(Relative_distance,Reference_m, Front_speed, Speed_set, AEB_range)
close_flag = 0;
Diff = Relative_distance - (Reference_m + AEB_range);
section = Reference_m/2;   % Section into two part

if Diff>30
    cmd = Speed_set;
elseif Diff>2 && Diff<=30
    cmd = Front_speed + 1*(Diff-3);
elseif Diff<=2 && Diff>0
    cmd = Front_speed;
elseif Diff<=0 && Diff>(-section)
    if Front_speed <2
        cmd = 0;
    else
        cmd = Front_speed + (Diff/section) *(Front_speed/3);
    end
elseif  Diff<=(-section)
    if Front_speed <2
        cmd = 0;
    else
        cmd = (2/3)*Front_speed + ((Diff+section)/section) * ((2/3)*Front_speed);
    end
    close_flag = 1;
else  % Unexpected situation
    cmd = 0;
end

if cmd>Speed_set
    cmd = Speed_set;
elseif cmd<0
    cmd = 0;
end

== matlab function bus_roadtest_v3/Speed_profile/High level controller/ACC/Filter ==
  data: u input; y output
function y = fcn(u)

if u>50
    u = 50;
elseif u<0
    u = 0;
end

y = u;
